simulink model "Simulation_2_model"  (R2017b)
settings: Solver=ode23tb  StartTime=0.0  StopTime=1  MaxStep=1e-6  RelTol=1e-3
values from neighbouring files (symbols this model uses):
  fs = 25000    [Simulation_1_code.m]    (also in Simulation_2_code.m)
  Jm = 0.02    [Simulation_1_code.m]    (also in Simulation_2_code.m)
  Ki_w = 1.5    [Simulation_2_code.m]
  Kp_w = 10    [Simulation_2_code.m]
  kt = 0.5    [Simulation_1_code.m]    (also in Simulation_2_code.m)
  La = 1.5e-3    (= 0.0015)    [Simulation_1_code.m]    (also in Simulation_2_code.m)
  Ra = 0.35    [Simulation_1_code.m]    (also in Simulation_2_code.m)
  Tf = 90    [Simulation_2_code.m]
  Ti = 30    [Simulation_2_code.m]
  Ttime = .5    (= 0.5)    [Simulation_2_code.m]
  Vdc = 200    [Simulation_1_code.m]    (also in Simulation_2_code.m)
  w_ref = 1500*((2*pi)/60)    (= 157.079632679)    [Simulation_2_code.m]
libraries: powerlib x9, simulink x2
settings Model: Creator=Jess  LastModifiedBy=Andrew McCullough

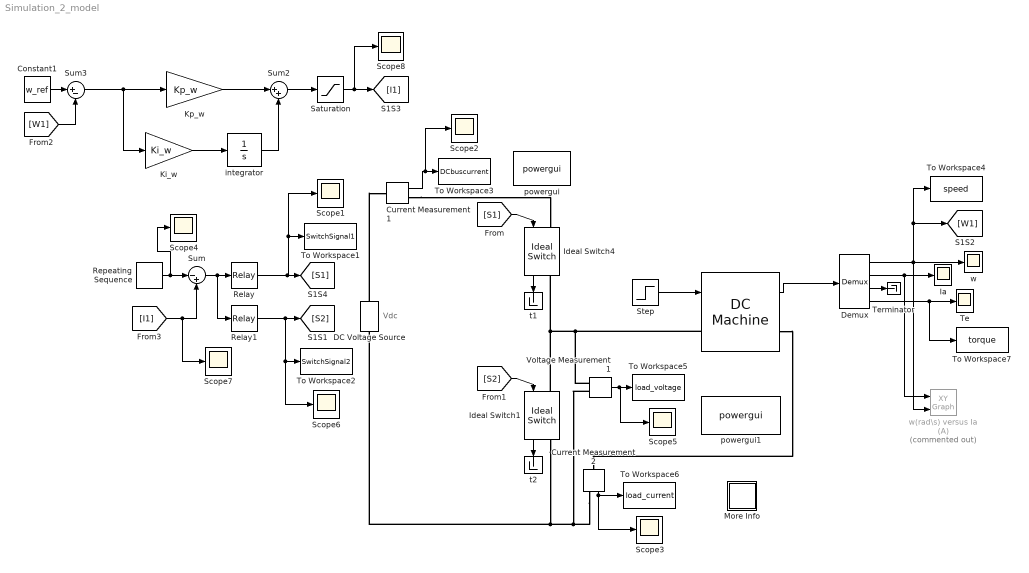
== system Simulation_2_model ==
  note: Vdc
  " " : powerlib/Machines/DC Machine  PresetModel=No  MechanicalLoad=Torque TL  FieldType=Permanent magnet  ShowDetailedParameters=on  MeasurementBus=off  RLa=[ Ra La]  RLf="[ 240  120]"  Laf=1.8  MachineConstant=Torque constant (N.m/A)  Ke=1.8  Kt=kt  J=Jm  Bm=0  Tf=0  w0=w_ref  Ifinit=1  TsPowergui=0  TsBlock=-1
      settings: AttributesFormatString=\n
  Constant1 : Constant  Value=w_ref
  Current Measurement1 : powerlib/Measurements/Current Measurement  PhasorSimulation=off  OutputType=Complex  PSBequivalent=0
  Current Measurement2 : powerlib/Measurements/Current Measurement  PhasorSimulation=off  OutputType=Complex  PSBequivalent=0
  DC Voltage Source : powerlib/Electrical Sources/DC Voltage Source  Amplitude=Vdc  Measurements=None
  Demux : Demux
  Ia : Scope
  Ideal Switch1 : powerlib/Power Electronics/Ideal Switch  Ron=0.001  Lon=0  IC=0  Rs=1e5  Cs=inf  Measurements=on
  Ideal Switch4 : powerlib/Power Electronics/Ideal Switch  Ron=0.001  Lon=0  IC=0  Rs=1e5  Cs=inf  Measurements=on
  Ki_w : Gain  Gain=Ki_w
  Kp_w : Gain  Gain=Kp_w
  More Info : Subsystem
      settings: OpenFcn=showdemo(bdroot(gcb))
      mask Display: disp('?')
  Relay : Relay
  Relay1 : Relay  OnOutputValue=0  OffOutputValue=1
  Repeating Sequence : simulink/Sources/Repeating Sequence  rep_seq_t=[0 0.5/fs 1/fs]  rep_seq_y=[0 1 0]
  Saturation : Saturate  UpperLimit=1  LowerLimit=0
  Scope{1..8} (8 alike) : Scope
  Step : Step  Time=Ttime  Before=Ti  After=Tf  SampleTime=0
  Sum : Sum  Inputs=|-+
  Sum2 : Sum  Inputs=|++
  Sum3 : Sum  Inputs=|+-
  Te : Scope
  Terminator : Terminator
  To Workspace1 : ToWorkspace  VariableName=SwitchSignal1  SaveFormat=Timeseries  SampleTime=-1
  To Workspace2 : ToWorkspace  VariableName=SwitchSignal2  SaveFormat=Timeseries  SampleTime=-1
  To Workspace3 : ToWorkspace  VariableName=DCbuscurrent  SaveFormat=Structure With Time  SampleTime=-1
  To Workspace4 : ToWorkspace  VariableName=speed  SaveFormat=Timeseries  SampleTime=-1
  To Workspace5 : ToWorkspace  VariableName=load_voltage  SaveFormat=Timeseries  SampleTime=-1
  To Workspace6 : ToWorkspace  VariableName=load_current  SaveFormat=Timeseries  SampleTime=-1
  To Workspace7 : ToWorkspace  VariableName=torque  SaveFormat=Timeseries  SampleTime=-1
  Voltage Measurement1 : powerlib/Measurements/Voltage Measurement  PhasorSimulation=off  OutputType=Complex  PSBequivalent=0
  integrator : Integrator  LimitOutput=on  UpperSaturationLimit=+5  LowerSaturationLimit=-5
  powergui : powerlib/powergui  Priority=1  SimulationMode=Continuous  SampleTime=50e-6  frequency=60  Iterations=50  frequencyindice=0  Pbase=100e6  ErrMax=1e-4  UnitsV=kV  UnitsW=MW  buscounter=0  FunctionMessages=off  echomessages=off  EnableUseOfTLC=off  CurrentSourceSwitches=off  DisableSnubberDevices=off  DisableRonSwitches=off  DisableVfSwitches=off  DisplayEquations=off  SolverType=Tustin/Backward Euler (TBE)  Interpol=off  ExternalGateDelay=off  methode=off  Ts=100  x0status=blocks  SPID=on  SwTol=0  HookPort=off  RestoreLinks=warning  ResistiveCurrentMeasurement=off  Frange=[0:2:500]  Ylog=off  Xlog=on  ShowGrid=off  save=off  variable=ZData  structure=voltage  ZoomFFT=off  StartTime=0.0  cycles=10  DisplayStyle=1  fundamental=100  FreqAxis=off  MaxFrequency=1000  frequencyindicesteady=1  RmsSteady=1  display=off
  powergui1 : powerlib/powergui  Priority=2  SimulationMode=Continuous  SampleTime=0  frequency=60  Iterations=50  frequencyindice=0  Pbase=100e6  ErrMax=1e-4  UnitsV=kV  UnitsW=MW  buscounter=0  FunctionMessages=off  echomessages=off  EnableUseOfTLC=off  CurrentSourceSwitches=off  DisableSnubberDevices=on  DisableRonSwitches=off  DisableVfSwitches=off  DisplayEquations=off  SolverType=Tustin  Interpol=off  ExternalGateDelay=off  methode=off  Ts=0  x0status=blocks  SPID=on  SwTol=0  HookPort=off  RestoreLinks=warning  ResistiveCurrentMeasurement=off  Frange=logspace(0,3,50)  Ylog=off  Xlog=off  ShowGrid=off  save=off  variable=ZData  structure=0  ZoomFFT=on  StartTime=0.0  cycles=1  DisplayStyle=off  fundamental=60  FreqAxis=off  MaxFrequency=1000  frequencyindicesteady=1  RmsSteady=1  display=off
  t1 : Terminator
  t2 : Terminator
  w : Scope
  w(rad\s) versus Ia (A) : simulink/Sinks/XY Graph  Commented=on  xmin=0  xmax=40  ymin=0  ymax=140  st=-1
  wires:
  [S1] -> Ideal Switch4/1
  Current Measurement1/1 -> Scope2/1, To Workspace3/1
  Relay/1 -> [S1], To Workspace1/1, Scope1/1
  [S2] -> Ideal Switch1/1
  Ideal Switch1/1 -> t2/1
  Ideal Switch4/1 -> t1/1
  Current Measurement2/1 -> To Workspace6/1, Scope3/1
  Repeating Sequence/1 -> Scope4/1, Sum/1
  Sum/1 -> Relay1/1, Relay/1
  Relay1/1 -> To Workspace2/1, Scope6/1, [S2]
  Voltage Measurement1/1 -> Scope5/1, To Workspace5/1
  Demux/1 -> To Workspace4/1, [W1], w/1, w(rad\s) versus Ia (A)/2
  Demux/2 -> Ia/1, w(rad\s) versus Ia (A)/1
  Demux/4 -> To Workspace7/1, Te/1
  " "/1 -> Demux/1
  Demux/3 -> Terminator/1
  Step/1 -> " "/1
  [W1] -> Sum3/2
  Sum3/1 -> Ki_w/1, Kp_w/1
  Ki_w/1 -> integrator/1
  integrator/1 -> Sum2/2
  Kp_w/1 -> Sum2/1
  Constant1/1 -> Sum3/1
  [I1] -> Scope7/1, Sum/2
  Sum2/1 -> Saturation/1
  Saturation/1 -> Scope8/1, [I1]
  connections:
  DC Voltage Source/RConn1 -- Current Measurement1/LConn1
  " "/LConn1 -- Voltage Measurement1/LConn1 -- Ideal Switch1/LConn1 -- Ideal Switch4/RConn1
  Current Measurement2/RConn1 -- Voltage Measurement1/LConn2 -- Ideal Switch1/RConn1 -- DC Voltage Source/LConn1
  Current Measurement1/RConn1 -- Ideal Switch4/LConn1
  " "/RConn1 -- Current Measurement2/LConn1

== system Simulation_2_model/More Info ==
